simulink model "Emidemiemodell"  (R2020b)
settings: Solver=VariableStepAuto  StartTime=0.0  StopTime=1000  RelTol=1e-3
undefined symbols (not defined in the file or in its folder): parSys
settings Model: Creator=paul  LastModifiedBy=Armin Wessel

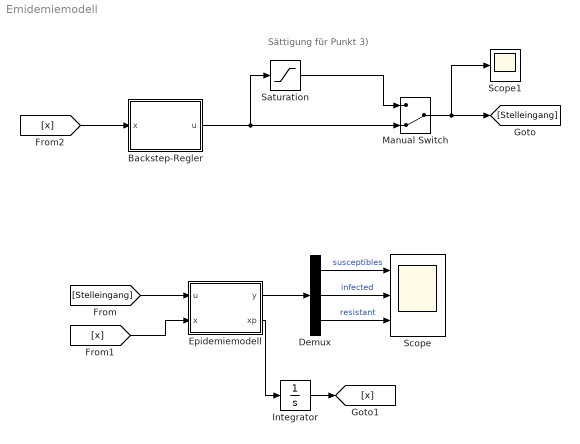
== system Emidemiemodell ==
  note: Sättigung für Punkt 3)
  Backstep-Regler : MATLAB Function  TreatAsAtomicUnit=on
  Demux : Demux  Outputs=3
  Epidemiemodell : MATLAB Function  TreatAsAtomicUnit=on
  Integrator : Integrator  InitialCondition=[parSys.i_0,parSys.r_0]
  Manual Switch : ManualSwitch  CurrentSetting=0
  Saturation : Saturate  UpperLimit=0.1  LowerLimit=0
  Scope : Scope  NumInputPorts=3
  Scope1 : Scope
  wires:
  [Stelleingang] -> Epidemiemodell/1(u)
  Demux/1 -> Scope/1  "susceptibles"
  Epidemiemodell/1(y) -> Demux/1
  Demux/2 -> Scope/2  "infected"
  Demux/3 -> Scope/3  "resistant"
  Epidemiemodell/2(xp) -> Integrator/1
  [x] -> Epidemiemodell/2(x)
  [x] -> Backstep-Regler/1(x)
  Backstep-Regler/1(u) -> Saturation/1, Manual Switch/2
  Manual Switch/1 -> Scope1/1, [Stelleingang]
  Integrator/1 -> [x]
  Saturation/1 -> Manual Switch/1

== matlab function Emidemiemodell/Backstep-Regler ==
  data: x input; u output; parSys parameter
function u = fcn(x,parSys)
% Input
i = x(1);
r = x(2);

% Par structure
par_beta = parSys.beta;
par_gamma = parSys.gamma;
par_delta = parSys.delta;

c1 = parSys.c1;
c2 = parSys.c2;
c = parSys.c;


%u = (i * (r - 1) * par_beta ^ 2 + ((-i - r + 2) * k1 + par_delta * r) * par_beta - 2 * k1 * par_gamma) / par_beta;
%u = ((-0.98e0 + r) * i * par_beta ^ 2 + ((-0.1e1 * i - 0.1e1 * r + 0.2e1) * k1 + par_delta * r) * par_beta - 0.2e1 * k1 * par_gamma) / par_beta;
u = -c2 * (r - 0.1e1 + 0.2e-1 * exp(log(i) + 0.3912023005e1) + par_gamma / par_beta - c1 * (log(i) + 0.3912023005e1) / par_beta) - 0.2e-1 * par_gamma * exp(log(i) + 0.3912023005e1) + par_delta * r + 0.5000000000e2 * (-0.2e-1 * exp(log(i) + 0.3912023005e1) + c1 / par_beta) * (0.2e-1 * par_beta * exp(log(i) + 0.3912023005e1) * (0.1e1 - 0.2e-1 * exp(log(i) + 0.3912023005e1) - r) - 0.2e-1 * par_gamma * exp(log(i) + 0.3912023005e1)) / exp(log(i) + 0.3912023005e1) + 0.1e1 / c * par_beta * (log(i) + 0.3912023005e1);

== matlab function Emidemiemodell/Epidemiemodell ==
  data: u input; y output; x input; xp output; parSys parameter
function [y,xp]= fcn(u,x, parSys)

xp = zeros(2,1);
y = zeros(3,1);
% Parameter holen
beta = parSys.beta;
gamma = parSys.gamma;
delta = parSys.delta;


xp(1) = beta*x(1)*(1-x(1)-x(2))-gamma*x(1); % x(1) = i
xp(2) = gamma*x(1)-delta*x(2)+u;

y(1) = 1-x(1)-x(2);
y(2) = x(1);
y(3) = x(2);
